simulink library "Drone_SISO_Subsystem"  (R2025b)
settings: Solver=VariableStepAuto  StartTime=0.0  StopTime=10.0  RelTol=1e-3
libraries: Drone_MIMO_Simple_Model x1
settings Model: Creator=Alek  LastModifiedBy=Alek

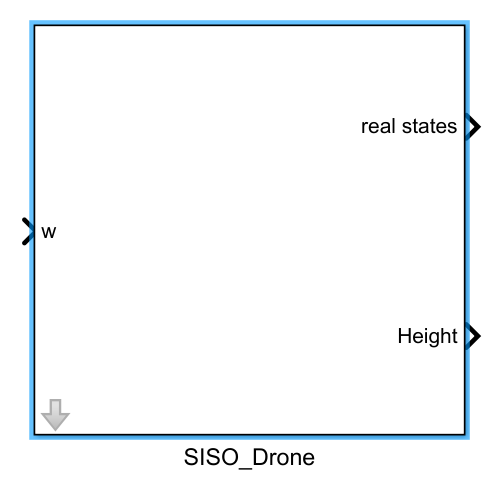
[thumbnail: Simulink's stored preview of the top-level diagram]
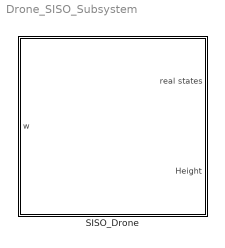
== system Drone_SISO_Subsystem ==
  SISO_Drone : Subsystem  mask{kf=1e-5, m=0.5, l=1e-2, I=6.6666e-5}
      mask prompts: kf "Thrust Coefficient"; m "Mass"; l "Arm Length"; I "Moment Of Intertia"

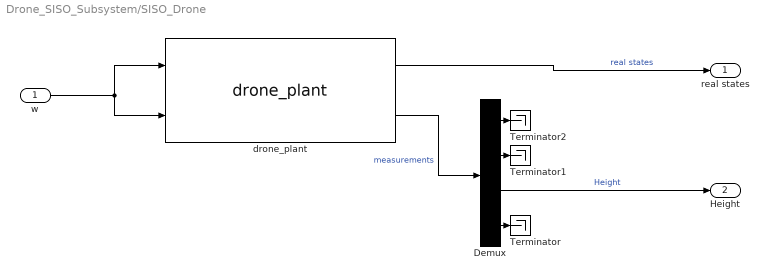
== system Drone_SISO_Subsystem/SISO_Drone ==
  w : Inport
  Demux : Demux
  Terminator : Terminator
  Terminator1 : Terminator
  Terminator2 : Terminator
  drone_plant : Drone_MIMO_Simple_Model/drone_plant  kf=kf  m=m  l=l  Irod=I
      settings: SourceProductName=DroneLibrary
  real states : Outport
  Height : Outport  Port=2  PortDimensions=1  SampleTime=1
  wires:
  w/1 -> drone_plant/1, drone_plant/2
  drone_plant/2 -> Demux/1  "measurements"
  Demux/2 -> Terminator1/1
  Demux/3 -> Height/1  "Height"
  Demux/1 -> Terminator2/1
  Demux/4 -> Terminator/1
  drone_plant/1 -> real states/1  "real states"
